simulink model "new_nncACCsystem_4_50"  (R2021a)
settings: Solver=FixedStepAuto  StartTime=0.0  StopTime=T  RelTol=1e-3
undefined symbols (not defined in the file): t_gap, Ts, v0_ego, v0_lead, v_set, x0_ego, x0_lead
libraries: neural x206
(part 11 of 11)

== system new_nncACCsystem_4_50/Feed-Forward Neural Network/Layer 5/Delays 1 ==
  "p{5}" : Inport  PortDimensions=50
      mask Display: e = 0.06;c1 = [120 230 180]/255;c2 = ([120 230 180]+0)/(256+128);c3 = ([120 230 180]+128)/(256+128);patch([0 1 1 0],[0 0 1 1],c1);patch([0 1 1 1-e 1-e 0+e],[0 0 1 1-e 0+e 0+e],c2);patch([0 0 1 1-e 0+e 0+e],[0 1 1 1-e 1-e 0+e],c3);plot([0 1 1 0 0],[0 0 1 1 0]);
  mux : Mux  Inputs=1
      mask Display: e = 0.06;c1 = [120 150 230]/255;c2 = ([120 150 230]+0)/383;c3 = ([120 150 230]+128)/383;patch([0 1 1 0],[0 0 1 1],c1);patch([0 1 1 1-e 1-e 0+e],[0 0 1 1-e 0+e 0+e],c2);patch([0 0 1 1-e 0+e 0+e],[0 1 1 1-e 1-e 0+e],c3);plot([0 1 1 0 0],[0 0 1 1 0]);disp('Mux')
  "pd{5,4}" : Outport
      mask Display: e = 0.06;c1 = [120 230 180]/255;c2 = ([120 230 180]+0)/(256+128);c3 = ([120 230 180]+128)/(256+128);patch([0 1 1 0],[0 0 1 1],c1);patch([0 1 1 1-e 1-e 0+e],[0 0 1 1-e 0+e 0+e],c2);patch([0 0 1 1-e 0+e 0+e],[0 1 1 1-e 1-e 0+e],c3);plot([0 1 1 0 0],[0 0 1 1 0]);
  wires:
  "p{5}"/1 -> mux/1
  mux/1 -> "pd{5,4}"/1

== system new_nncACCsystem_4_50/Feed-Forward Neural Network/Layer 5/LW{5,4} ==
  "ad{5,4}" : Inport  PortDimensions=50
      mask Display: e = 0.06;c1 = [120 230 180]/255;c2 = ([120 230 180]+0)/(256+128);c3 = ([120 230 180]+128)/(256+128);patch([0 1 1 0],[0 0 1 1],c1);patch([0 1 1 1-e 1-e 0+e],[0 0 1 1-e 0+e 0+e],c2);patch([0 0 1 1-e 0+e 0+e],[0 1 1 1-e 1-e 0+e],c3);plot([0 1 1 0 0],[0 0 1 1 0]);
  "IW{5,4}(1,:)'" : Constant  Value=[0.38759828050434019797165774434688501060009002685546875;-0.3075219555673263105433079545036889612674713134765625;-0.0153138181681681424806118485548722674138844013214111328125;-0.6412079453251251504042329543153755366802215576171875;0.7928410496461333334394794292165897786617279052734375;0.609017552404527151566071552224457263946533203125;-0.64843436097298823295176362080383114516735076904296875;-0.1994028373608804916017334107891656458377838134765625;0.83748274751696183404447992870700545608997344970703125;-0.484292818768689070640931504385662265121936798095703125;-0.181663741035503589760224940619082190096378326416015625;-0.92747174629596684791721372675965540111064910888671875;-0.96205783726095284169588239819859154522418975830078125;0.76826850988010242371473168532247655093669891357421875;0.3970028385512540669566305950866080820560455322265625;-0.6014566916400549967391953032347373664379119873046875;0.276052746200821375044398564568837173283100128173828125;-0.7032530380507953093882633766042999923229217529296875;0.8490335532649131433657885281718336045742034912109375;-0.00965973194881899858976748163286174531094729900360107421875;-0.5804614860588148683717690801131539046764373779296875;-0.339377234494642798789953985760803334414958953857421875;0.1115453173116549567822630706359632313251495361328125;0.358807507862387742303411641842103563249111175537109375;0.007904888754092898039971260004676878452301025390625;0.463699948195857303279154848496546037495136260986328125;0.767362214732545400153185255476273596286773681640625;-0.27987824453678189495775541217881254851818084716796875;-0.59315992208557799525436848853132687509059906005859375;0.5286601386597311602599802426993846893310546875;-0.96428714358694822550432945718057453632354736328125;0.1650415295214242572541252229711972177028656005859375;-0.40236027206437408043626646758639253675937652587890625;0.301669620069009380980418200124404393136501312255859375;0.39279787121216980239069016533903777599334716796875;0.391971054861243894951172705987119115889072418212890625;-0.605245261904915565764895291067659854888916015625;-0.12651170183679372183149780539679341018199920654296875;-0.836649505666742232534716094960458576679229736328125;0.24687610665629999839865149624529294669628143310546875;-0.1616835205137980846501477572019211947917938232421875;0.2060349468751774271169097119127400219440460205078125;-0.4898289350080589077407466902513988316059112548828125;0.6177615612048528159760962807922624051570892333984375;-0.3933731322621516479642878039157949388027191162109375;-0.350940255028392211755772223114036023616790771484375;-0.31081513135482696785771850045421160757541656494140625;0.6602177997017031341187021098448894917964935302734375;-0.947685882785339384071221502381376922130584716796875;-0.6605981173973558551182350129238329827785491943359375]
      mask Display: e = 0.06;c1 = [120 150 230]/255;c2 = ([120 150 230]+0)/383;c3 = ([120 150 230]+128)/383;patch([0 1 1 0],[0 0 1 1],c1);patch([0 1 1 1-e 1-e 0+e],[0 0 1 1-e 0+e 0+e],c2);patch([0 0 1 1-e 0+e 0+e],[0 1 1 1-e 1-e 0+e],c3);plot([0 1 1 0 0],[0 0 1 1 0]);disp('weights');
  Mux : Mux  Inputs=1
      mask Display: e = 0.06;c1 = [120 150 230]/255;c2 = ([120 150 230]+0)/383;c3 = ([120 150 230]+128)/383;patch([0 1 1 0],[0 0 1 1],c1);patch([0 1 1 1-e 1-e 0+e],[0 0 1 1-e 0+e 0+e],c2);patch([0 0 1 1-e 0+e 0+e],[0 1 1 1-e 1-e 0+e],c3);plot([0 1 1 0 0],[0 0 1 1 0]);disp('Mux');
  dotprod1 : neural/Weight Functions/dotprod
  "lz{5,4}" : Outport
      mask Display: e = 0.06;c1 = [120 230 180]/255;c2 = ([120 230 180]+0)/(256+128);c3 = ([120 230 180]+128)/(256+128);patch([0 1 1 0],[0 0 1 1],c1);patch([0 1 1 1-e 1-e 0+e],[0 0 1 1-e 0+e 0+e],c2);patch([0 0 1 1-e 0+e 0+e],[0 1 1 1-e 1-e 0+e],c3);plot([0 1 1 0 0],[0 0 1 1 0]);
  wires:
  "IW{5,4}(1,:)'"/1 -> dotprod1/1
  "ad{5,4}"/1 -> dotprod1/2
  dotprod1/1 -> Mux/1
  Mux/1 -> "lz{5,4}"/1
